simulink model "foc_dq_closed_loop_autogen"  (R2024a)
settings: Solver=FixedStepDiscrete  StartTime=0.0  StopTime=0.05  FixedStep=5e-05  RelTol=1e-3
settings Model: Creator=黄钟锐  LastModifiedBy=黄钟锐
settings SFSimCC: SimCustomHeaderCode="#include \"sim/foc_sim.h\""
settings SFSimCC: SimUserSources=|
  | src\sim\foc_sim.c
  | src\control\current_controller.c
  | src\foc\foc_math.c
  | src\foc\svpwm.c
settings SFSimCC: SimUserIncludeDirs=|
  | include
  | src
  | src\sim
  | src\control
  | src\foc

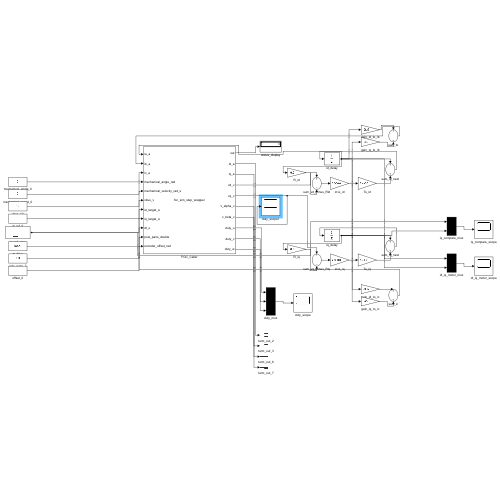
[thumbnail: Simulink's stored preview of the top-level diagram]
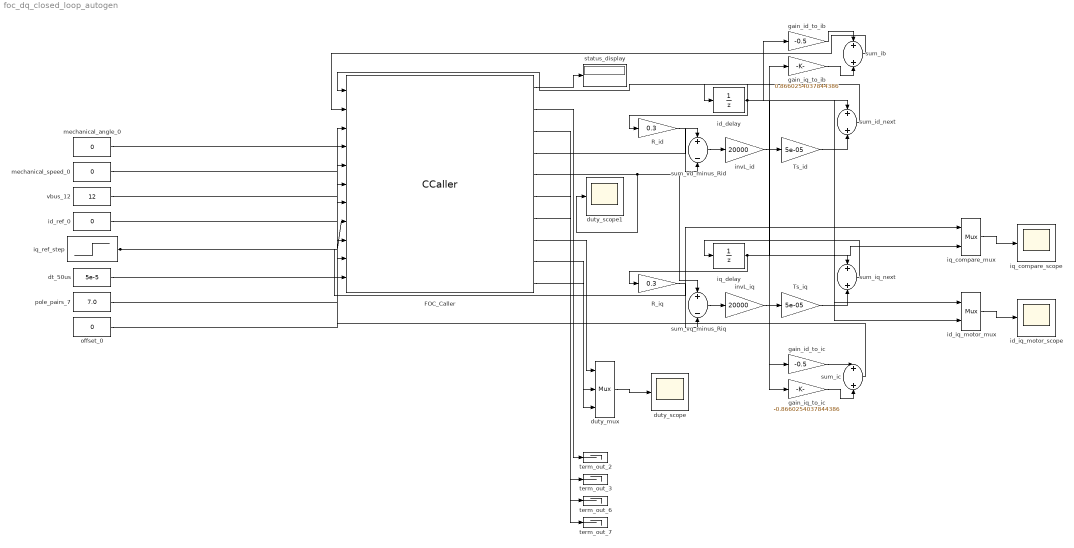
== system foc_dq_closed_loop_autogen ==
  FOC_Caller : CCaller  FunctionName=foc_sim_step_wrapper  PortSpecificationStruct="%)30     .    &\"0   8    (     @         %    \"    !4    !     0         %  0 \"0    $    _    07)G3F%M90  4&]R=$YA;64 4V-O<&4     26YD97@     5'EP90      4VEZ90      27-';&]B86P   X    P    !@    @    $          4    (     0    ,    !         !   P!O=70 #@   #     &    \"     0         !0    @    !     P    $         $  # &]U=  .    .     8    (    !          %    \"     $    &     0         0  ...(+12085 chars)"  SampleTime=5e-05
  R_id : Gain  Gain=0.3
  R_iq : Gain  Gain=0.3
  Ts_id : Gain  Gain=5e-05
  Ts_iq : Gain  Gain=5e-05
  dt_50us : Constant  Value=5e-5  SampleTime=5e-5
  duty_mux : Mux  Inputs=3
  duty_scope : Scope
  duty_scope1 : Scope
  gain_id_to_ib : Gain  Gain=-0.5
  gain_id_to_ic : Gain  Gain=-0.5
  gain_iq_to_ib : Gain  Gain=0.8660254037844386
  gain_iq_to_ic : Gain  Gain=-0.8660254037844386
  id_delay : UnitDelay  SampleTime=5e-05  HasFrameUpgradeWarning=on
  id_iq_motor_mux : Mux  Inputs=2
  id_iq_motor_scope : Scope
  id_ref_0 : Constant  Value=0  SampleTime=5e-5
  invL_id : Gain  Gain=20000
  invL_iq : Gain  Gain=20000
  iq_compare_mux : Mux  Inputs=2
  iq_compare_scope : Scope
  iq_delay : UnitDelay  SampleTime=5e-05  HasFrameUpgradeWarning=on
  iq_ref_step : Step  Time=0.005  After=0.5  SampleTime=5e-5
  mechanical_angle_0 : Constant  Value=0  SampleTime=5e-5
  mechanical_speed_0 : Constant  Value=0  SampleTime=5e-5
  offset_0 : Constant  Value=0  SampleTime=5e-5
  pole_pairs_7 : Constant  Value=7.0  SampleTime=5e-5
  status_display : Display
  sum_ib : Sum
  sum_ic : Sum
  sum_id_next : Sum
  sum_iq_next : Sum
  sum_vd_minus_Rid : Sum  Inputs=+-
  sum_vq_minus_Riq : Sum  Inputs=+-
  term_out_{2..3,6..7} (4 alike) : Terminator
  vbus_12 : Constant  Value=12  SampleTime=5e-5
  wires:
  id_delay/1 -> FOC_Caller/1, R_id/1, sum_id_next/1, gain_id_to_ib/1, gain_id_to_ic/1, id_iq_motor_mux/1
  sum_ib/1 -> FOC_Caller/2
  sum_ic/1 -> FOC_Caller/3
  mechanical_angle_0/1 -> FOC_Caller/4
  mechanical_speed_0/1 -> FOC_Caller/5
  vbus_12/1 -> FOC_Caller/6
  id_ref_0/1 -> FOC_Caller/7
  iq_ref_step/1 -> FOC_Caller/8, iq_compare_mux/1
  dt_50us/1 -> FOC_Caller/9
  pole_pairs_7/1 -> FOC_Caller/10
  offset_0/1 -> FOC_Caller/11
  R_id/1 -> sum_vd_minus_Rid/2
  sum_vd_minus_Rid/1 -> invL_id/1
  invL_id/1 -> Ts_id/1
  Ts_id/1 -> sum_id_next/2
  sum_id_next/1 -> id_delay/1
  FOC_Caller/5 -> duty_scope1/1, sum_vq_minus_Riq/1
  iq_delay/1 -> R_iq/1, sum_iq_next/1, gain_iq_to_ib/1, gain_iq_to_ic/1, iq_compare_mux/2, id_iq_motor_mux/2
  R_iq/1 -> sum_vq_minus_Riq/2
  sum_vq_minus_Riq/1 -> invL_iq/1
  invL_iq/1 -> Ts_iq/1
  Ts_iq/1 -> sum_iq_next/2
  sum_iq_next/1 -> iq_delay/1
  gain_id_to_ib/1 -> sum_ib/1
  gain_iq_to_ib/1 -> sum_ib/2
  gain_id_to_ic/1 -> sum_ic/1
  gain_iq_to_ic/1 -> sum_ic/2
  FOC_Caller/1 -> status_display/1
  FOC_Caller/8 -> duty_mux/1
  FOC_Caller/9 -> duty_mux/2
  FOC_Caller/10 -> duty_mux/3
  duty_mux/1 -> duty_scope/1
  iq_compare_mux/1 -> iq_compare_scope/1
  id_iq_motor_mux/1 -> id_iq_motor_scope/1
  FOC_Caller/2 -> term_out_2/1
  FOC_Caller/3 -> term_out_3/1
  FOC_Caller/6 -> term_out_6/1
  FOC_Caller/7 -> term_out_7/1
  FOC_Caller/4 -> sum_vd_minus_Rid/1
